simulink library "clock_lib"  (R2018b)
settings: Solver=VariableStepAuto  StartTime=0.0  StopTime=10.0  RelTol=1e-3
undefined symbols (not defined in the file or in its folder): simParams
settings Model: Creator=devantormey  LastModifiedBy=taylorreynolds

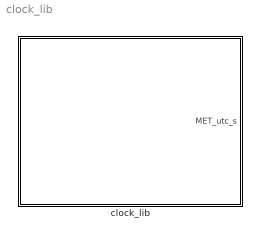
== system clock_lib ==
  clock_lib : Subsystem

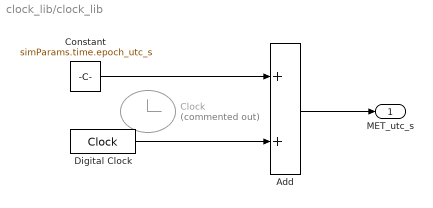
== system clock_lib/clock_lib ==
  Add : Sum
  Clock : Clock  Commented=on
  Constant : Constant  Value=simParams.time.epoch_utc_s
  Digital Clock : DigitalClock  SampleTime=simParams.sample_time_s
  MET_utc_s : Outport
  wires:
  Constant/1 -> Add/1
  Digital Clock/1 -> Add/2
  Add/1 -> MET_utc_s/1
